simulink subsystem "ControlObject"  (R2023a)
settings: Solver=VariableStepAuto  StartTime=0.0  StopTime=10.0  RelTol=1e-3
undefined symbols (not defined in the file): DemoControllers
settings Model: Creator=KozlovM  LastModifiedBy=Maxim

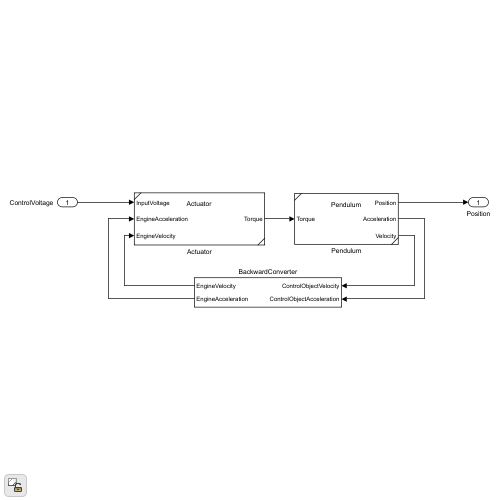
[thumbnail: Simulink's stored preview of the top-level diagram]
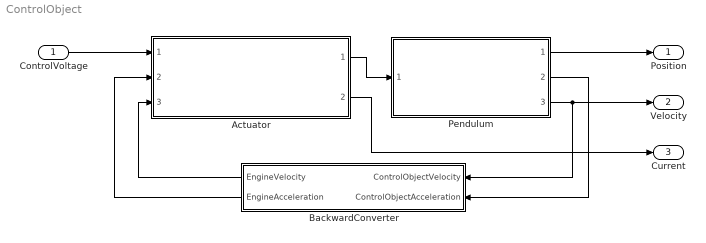
== system ControlObject ==
  ControlVoltage : Inport
  Actuator : Subsystem  ReferencedSubsystem=Actuator
  BackwardConverter : Subsystem
  Pendulum : Subsystem  ReferencedSubsystem=Pendulum
  Position : Outport
  Velocity : Outport  Port=2
  Current : Outport  Port=3
  wires:
  Pendulum/3 -> BackwardConverter/1(ControlObjectVelocity), Velocity/1
  Actuator/1 -> Pendulum/1
  Pendulum/2 -> BackwardConverter/2(ControlObjectAcceleration)
  BackwardConverter/2(EngineAcceleration) -> Actuator/2
  ControlVoltage/1 -> Actuator/1
  BackwardConverter/1(EngineVelocity) -> Actuator/3
  Actuator/2 -> Current/1
  Pendulum/1 -> Position/1

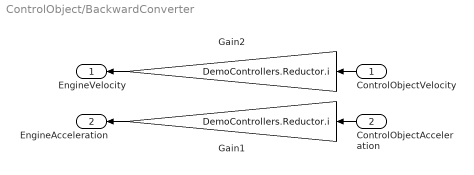
== system ControlObject/BackwardConverter ==
  ControlObjectVelocity : Inport
  ControlObjectAcceleration : Inport  Port=2
  Gain1 : Gain  Gain=DemoControllers.Reductor.i
  Gain2 : Gain  Gain=DemoControllers.Reductor.i
  EngineVelocity : Outport
  EngineAcceleration : Outport  Port=2
  wires:
  ControlObjectAcceleration/1 -> Gain1/1
  Gain2/1 -> EngineVelocity/1
  Gain1/1 -> EngineAcceleration/1
  ControlObjectVelocity/1 -> Gain2/1
